simulink subsystem "Longitudinal_Controller"  (R2020b)
settings: Solver=VariableStepAuto  StartTime=0.0  StopTime=10.0  RelTol=1e-3
undefined symbols (not defined in the file): Sim_Ts, Vehicle_id, Vehicles
libraries: mpcadaslib x1, simulink x1, pid_lib x1
settings Model: Creator=mustafa  LastModifiedBy=mustafa

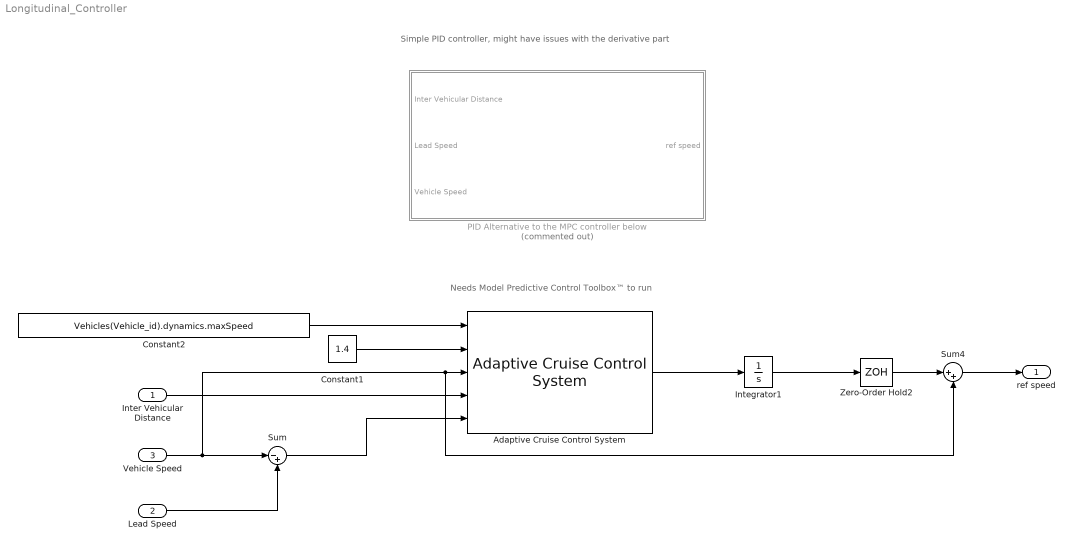
== system Longitudinal_Controller ==
  note: Needs Model Predictive Control Toolbox™ to run
  note: Simple PID controller, might have issues with the derivative part
  Inter Vehicular Distance : Inport
  Lead Speed : Inport  Port=2
  Vehicle Speed : Inport  Port=3
  Adaptive Cruise Control System : mpcadaslib/Adaptive Cruise Control System  EgoModel=tf(1,[1,0])  InitialEgoVelocity=0  DefaultSpacing=Vehicles(Vehicle_id).sensors.safeDistance  MaxVelocity=Vehicles(Vehicle_id).dynamics.maxSpeed  MinAcceleration=-3  amin_ext=off  MaxAcceleration=2  amax_ext=off  Ts=0.4  PredictionHorizon=5  ControllerBehavior=0.620  suboptimal=off  maxiter=10  datatypeopt=double  optmode=off  trackmode=off
  Constant1 : Constant  Value=1.4
  Constant2 : Constant  Value=Vehicles(Vehicle_id).dynamics.maxSpeed
  Integrator1 : Integrator  LimitOutput=on  UpperSaturationLimit=2  LowerSaturationLimit=-3
  PID Alternative to the MPC controller below : Subsystem  Commented=on
  Sum : Sum  Inputs=|-+
  Sum4 : Sum  Inputs=|++
  Zero-Order Hold2 : ZeroOrderHold  SampleTime=Sim_Ts
  ref speed : Outport  VectorParamsAs1DForOutWhenUnconnected=off
  wires:
  Vehicle Speed/1 -> Sum/1, Adaptive Cruise Control System/3, Sum4/2
  Lead Speed/1 -> Sum/2
  Inter Vehicular Distance/1 -> Adaptive Cruise Control System/4
  Sum/1 -> Adaptive Cruise Control System/5
  Constant1/1 -> Adaptive Cruise Control System/2
  Constant2/1 -> Adaptive Cruise Control System/1
  Adaptive Cruise Control System/1 -> Integrator1/1
  Integrator1/1 -> Zero-Order Hold2/1
  Zero-Order Hold2/1 -> Sum4/1
  Sum4/1 -> ref speed/1

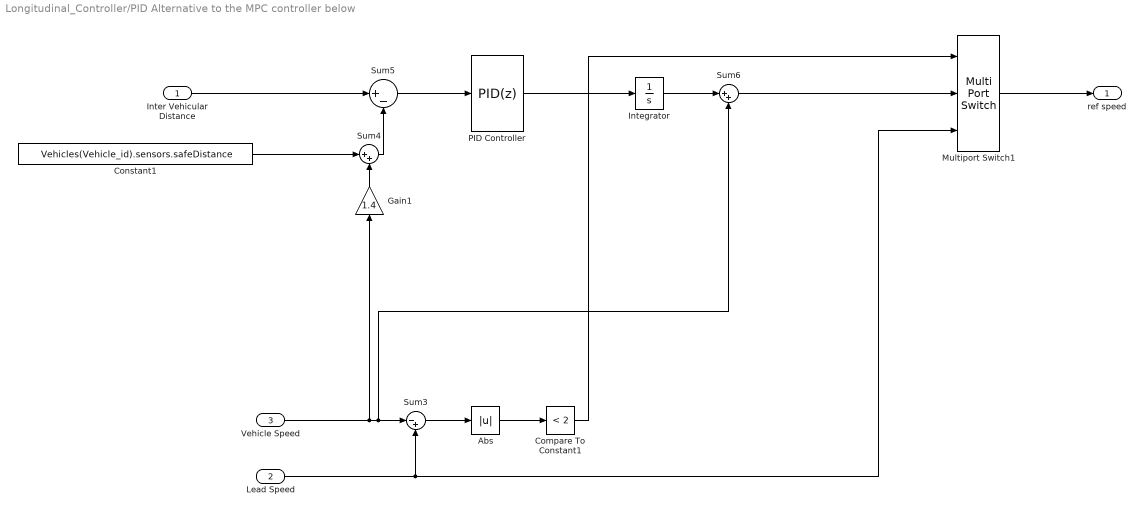
== system Longitudinal_Controller/PID Alternative to the MPC controller below ==
  Inter Vehicular Distance : Inport
  Lead Speed : Inport  Port=2
  Vehicle Speed : Inport  Port=3
  Abs : Abs
  Compare To Constant1 : simulink/Logic and Bit Operations/Compare To Constant  relop=<  const=2  OutDataTypeStr=uint8
  Constant1 : Constant  Value=Vehicles(Vehicle_id).sensors.safeDistance
  Gain1 : Gain  Gain=1.4
  Integrator : Integrator  LimitOutput=on  UpperSaturationLimit=2  LowerSaturationLimit=-3
  Multiport Switch1 : MultiPortSwitch  DataPortOrder=Zero-based contiguous  Inputs=2  zeroidx=on
  PID Controller : pid_lib/PID Controller  Controller=PID  Form=Parallel  TimeDomain=Discrete-time  UseExternalTs=off  SampleTime=0.02  IntegratorMethod=Forward Euler  FilterMethod=Forward Euler  ControllerParametersSource=internal  P=2  I=0.4  D=2  UseFilter=on  N=230  TunerSelectOption=Transfer Function Based (PID Tuner App)  InitialConditionSource=internal  InitialConditionForIntegrator=0  InitialConditionForFilter=0  DifferentiatorICPrevScaledInput=0  ExternalReset=none  TrackingMode=off  Kt=1  LimitOutput=on  SatLimitsSource=internal  UpperSaturationLimit=2  LowerSaturationLimit=-3  LinearizeAsGain=on  AntiWindupMode=none  Kb=1  POutMin=[]  POutMax=[]  IOutMin=[]  IOutMax=[]  DOutMin=[]  DOutMax=[]  NOutMin=[]  NOutMax=[]  SumOutMin=[]  SumOutMax=[]  SaturationOutMin=[]  SaturationOutMax=[]  PParamMin=[]  PParamMax=[]  IParamMin=[]  IParamMax=[]  DParamMin=[]  DParamMax=[]  NParamMin=[]  NParamMax=[]  KbParamMin=[]  KbParamMax=[]  KtParamMin=[]  KtParamMax=[]  KbOutMin=[]  KbOutMax=[]  KtOutMin=[]  KtOutMax=[]  IntegratorOutMin=[]  IntegratorOutMax=[]  FilterOutMin=[]  FilterOutMax=[]  SumI1OutMin=[]  SumI1OutMax=[]  SumI2OutMin=[]  SumI2OutMax=[]  SumI3OutMin=[]  SumI3OutMax=[]  SumI4OutMin=[]  SumI4OutMax=[]  SumDOutMin=[]  SumDOutMax=[]  DifferentiatorOutMin=[]  DifferentiatorOutMax=[]  FilterDiffOutCoefMin=[]  FilterDiffOutCoefMax=[]  ReciprocalOutMin=[]  ReciprocalOutMax=[]  SumDenOutMin=[]  SumDenOutMax=[]  SumNumOutMin=[]  SumNumOutMax=[]  DivideOutMin=[]  DivideOutMax=[]  UdiffTsProdOutMin=[]  UdiffTsProdOutMax=[]  NTsProdOutMin=[]  NTsProdOutMax=[]  UintegralTsProdOutMin=[]  UintegralTsProdOutMax=[]  UngainTsProdOutMin=[]  UngainTsProdOutMax=[]  IntegratorContinuousStateAttributes=''  IntegratorStateMustResolveToSignalObject=off  IntegratorRTWStateStorageClass=Auto  FilterContinuousStateAttributes=''  FilterStateMustResolveToSignalObject=off  FilterRTWStateStorageClass=Auto  ParallelPVariant=InternalParameters  IdealPVariant=Disabled  IVariant=InternalParameters  DVariant=InternalParameters  IntegratorVariant=Discrete  SatVariant=Enabled  AWVariant=Passthrough  PCopyVariant=Disabled  TRVariant=Disabled  FdbkBlocksVariant=Forward  IdealPFdbkVariant=Disabled  SatFdbkVariant=Disabled  DerivativeFilterVariant=ForwardEulerFilter  NVariant=InternalParameters  NCopyVariant=Disabled  FilterICVariant=InternalICsFilter  IntegratorICVariant=InternalICs  ExternalResetVariant=Disabled  TRSumVariant=Passthrough  SumFdbkVariant=Disabled  SumVariant=Sum_PID  TsampFilterVariant=InternalTs  TsampNgainVariant=Passthrough  TsampIntegralVariant=Passthrough  ExternalSaturationOutDataTypeStr=Inherit: Same as second input
  Sum3 : Sum  Inputs=|-+
  Sum4 : Sum  Inputs=|++
  Sum5 : Sum  Inputs=|+-
  Sum6 : Sum  Inputs=|++
  ref speed : Outport  VectorParamsAs1DForOutWhenUnconnected=off
  wires:
  Sum4/1 -> Sum5/2
  Sum5/1 -> PID Controller/1
  Sum3/1 -> Abs/1
  Sum6/1 -> Multiport Switch1/2
  Multiport Switch1/1 -> ref speed/1
  Compare To Constant1/1 -> Multiport Switch1/1
  Lead Speed/1 -> Sum3/2, Multiport Switch1/3
  Abs/1 -> Compare To Constant1/1
  Inter Vehicular Distance/1 -> Sum5/1
  Vehicle Speed/1 -> Gain1/1, Sum6/2, Sum3/1
  Constant1/1 -> Sum4/1
  Integrator/1 -> Sum6/1
  Gain1/1 -> Sum4/2
  PID Controller/1 -> Integrator/1
